simulink model "Exercise_2_2_1_Linear"  (R2021b)
settings: Solver=VariableStepAuto  StartTime=0.0  StopTime=simTime  RelTol=1e-3
values from neighbouring files (symbols this model uses):
  RPM = [0 1000 0 1000]    [Exercise_2_Workspace.mat]
  TakeStep = 1    [Exercise_2_Workspace.mat]
  uss = [11.0736172952 11.0736172952 11.0736172952 11.0736172952]    [Exercise_2_Workspace.mat]
  xss = [-1.12940484321e-22 -1.12940484321e-22 -1.12940484321e-22 -6.92906777586e-24 -7.18108347987e-24 -2.25889833838e-24 -2.12374037934e-26 -1.04079074138e-26 -1.12940484322e-22 -3.07253921614e-33 2.20405190779e-39 1.12940484322e-22]    [Exercise_2_Workspace.mat]
undefined symbols (not defined in the file or in its folder): Aa, Bb, Cc, Dd
settings Model: Creator=Wojciech  LastModifiedBy=tanzc

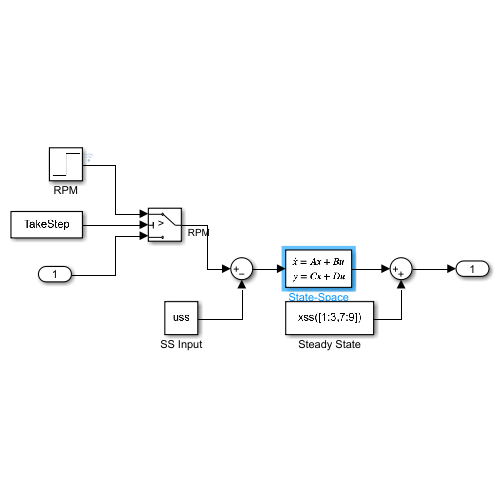
[thumbnail: Simulink's stored preview of the top-level diagram]
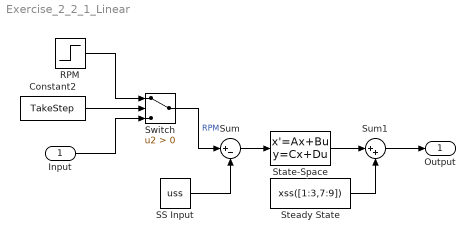
== system Exercise_2_2_1_Linear ==
  Input : Inport
  Constant2 : Constant  Value=TakeStep
  RPM : Step  Time=0  After=RPM  SampleTime=0
  SS Input : Constant  Value=uss  VectorParams1D=off
  State-Space : StateSpace  A=Aa  B=Bb  C=Cc  D=Dd  InitialCondition=xss
  Steady State : Constant  Value=xss([1:3,7:9])  VectorParams1D=off
  Sum : Sum  Inputs=|+-
  Sum1 : Sum  Inputs=|++
  Switch : Switch  Criteria=u2 > Threshold
  Output : Outport
  wires:
  SS Input/1 -> Sum/2
  State-Space/1 -> Sum1/1
  Sum1/1 -> Output/1
  Steady State/1 -> Sum1/2
  Sum/1 -> State-Space/1
  RPM/1 -> Switch/1
  Constant2/1 -> Switch/2
  Input/1 -> Switch/3
  Switch/1 -> Sum/1  "RPM"
